simulink model "Problem4"  (R2020b)
settings: Solver=VariableStepAuto  StartTime=0.0  StopTime=10.0  RelTol=1e-3
settings Model: Creator=HP  LastModifiedBy=HP

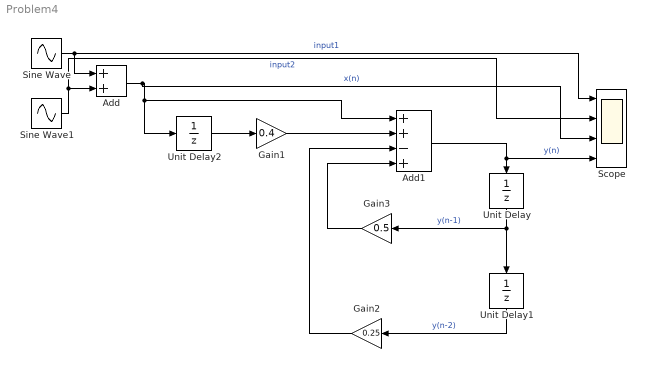
== system Problem4 ==
  Add : Sum
  Add1 : Sum  Inputs=++-+
  Gain1 : Gain  Gain=0.4
  Gain2 : Gain  Gain=0.25
  Gain3 : Gain  Gain=0.5
  Scope : Scope  NumInputPorts=4
  Sine Wave : Sin  SampleTime=0
  Sine Wave1 : Sin  Frequency=50  SampleTime=0
  Unit Delay : UnitDelay  SampleTime=-1  HasFrameUpgradeWarning=on
  Unit Delay1 : UnitDelay  SampleTime=-1  HasFrameUpgradeWarning=on
  Unit Delay2 : UnitDelay  SampleTime=-1  HasFrameUpgradeWarning=on
  wires:
  Sine Wave/1 -> Scope/1, Add/1  "input1"
  Sine Wave1/1 -> Scope/2, Add/2  "input2"
  Add/1 -> Scope/3, Add1/1, Unit Delay2/1  "x(n)"
  Gain1/1 -> Add1/2
  Unit Delay/1 -> Unit Delay1/1, Gain3/1  "y(n-1)"
  Gain3/1 -> Add1/4
  Gain2/1 -> Add1/3
  Unit Delay1/1 -> Gain2/1  "y(n-2)"
  Unit Delay2/1 -> Gain1/1
  Add1/1 -> Scope/4, Unit Delay/1  "y(n)"
